simulink model "ardupilot_sil_connector_example"  (R2022a)
settings: Solver=FixedStepAuto  StartTime=0.0  StopTime=inf  FixedStep=0.01  RelTol=1e-3
settings Model: Creator=kboychev  LastModifiedBy=kboychev
settings SolverCC: AlgebraicLoopSolver=TrustRegion
settings DataIOCC: ReturnWorkspaceOutputs=off
settings DebuggingCC: UnconnectedInputMsg=warning  UnconnectedOutputMsg=warning  UnconnectedLineMsg=warning  SFMachineParentedDataDiag=warning  ArithmeticOperatorsInVariantConditions=warning
settings SFSimCC: CustomCodeUndefinedFunction=UseInterfaceOnly

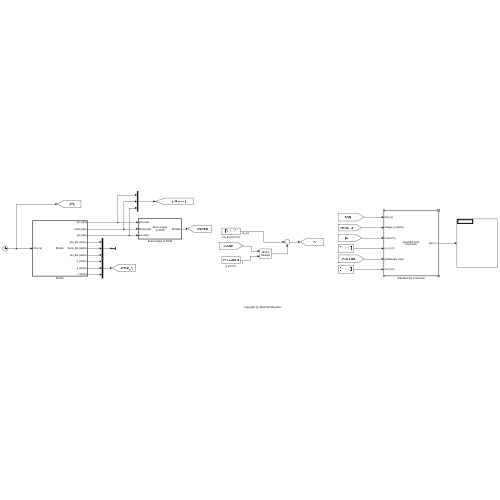
[thumbnail: Simulink's stored preview of the top-level diagram]
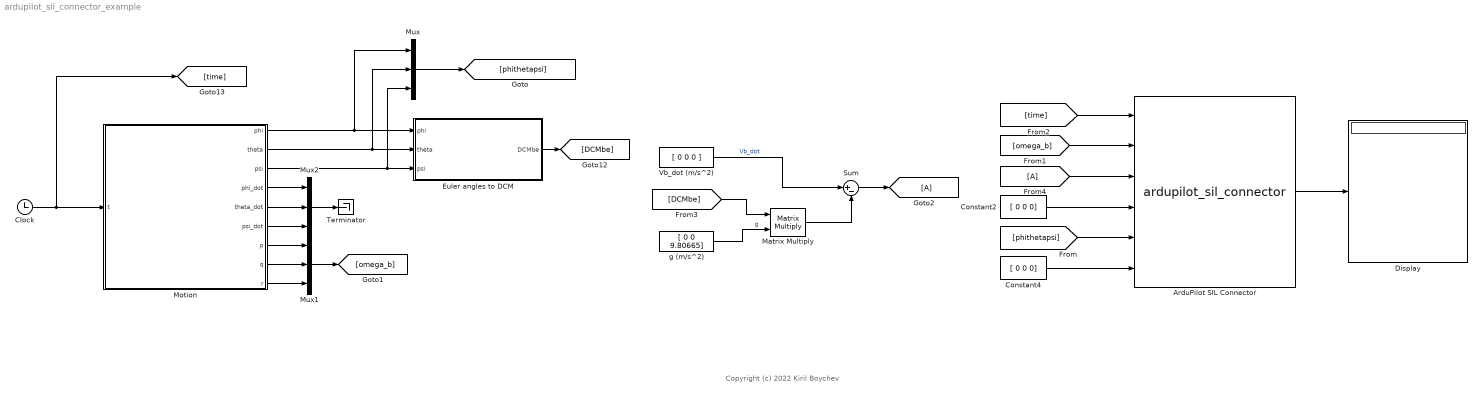
== system ardupilot_sil_connector_example ==
  note: Copyright (c) 2022 Kiril Boychev
  ArduPilot SIL Connector : S-Function  FunctionName=ardupilot_sil_connector  SFunctionDeploymentMode=off  EnableBusSupport=off
      mask Display:
      | fprintf('ArduPilot SITL\nConnector');
      | port_label('input', 1, 'time (s)');
      | port_label('input', 2, 'omega_b (rad/s)');
      | port_label('input', 3, 'A (m/s^2)');
      | port_label('input', 4, 'x y z (m)');
      | port_label('input', 5, 'phithetapsi (rad)');
      | port_label('input', 6, 'Vb (m/s)');
      | port_label('output', 1, 'pwm (-)');
  Clock : Clock
  Constant2 : Constant  Value=[ 0 0 0]
  Constant4 : Constant  Value=[ 0 0 0]
  Display : Display
  Euler angles to DCM : MATLAB Function  TreatAsAtomicUnit=on
  From4 : From
  Goto2 : Goto
  Matrix Multiply : Product  Multiplication=Matrix(*)
  Motion : MATLAB Function  TreatAsAtomicUnit=on
  Mux : Mux  Inputs=3
  Mux1 : Mux  Inputs=3
  Mux2 : Mux  Inputs=3
  Sum : Sum  Inputs=|+-
  Terminator : Terminator
  Vb_dot (m/s^2) : Constant  Value=[ 0 0 0 ]
  g (m/s^2) : Constant  Value=[ 0 0 9.80665]
  wires:
  ArduPilot SIL Connector/1 -> Display/1
  Constant2/1 -> ArduPilot SIL Connector/4
  [phithetapsi] -> ArduPilot SIL Connector/5
  [omega_b] -> ArduPilot SIL Connector/2
  [time] -> ArduPilot SIL Connector/1
  Motion/1(phi) -> Euler angles to DCM/1(phi), Mux/1
  Motion/3(psi) -> Mux/3, Euler angles to DCM/3(psi)
  Motion/2(theta) -> Mux/2, Euler angles to DCM/2(theta)
  Motion/7(p) -> Mux1/1
  Clock/1 -> [time], Motion/1(t)
  Mux/1 -> [phithetapsi]
  Mux1/1 -> [omega_b]
  Euler angles to DCM/1(DCMbe) -> [DCMbe]
  Motion/4(phi_dot) -> Mux2/1
  Motion/9(r) -> Mux1/3
  Mux2/1 -> Terminator/1
  Motion/5(theta_dot) -> Mux2/2
  Motion/8(q) -> Mux1/2
  Motion/6(psi_dot) -> Mux2/3
  Constant4/1 -> ArduPilot SIL Connector/6
  [DCMbe] -> Matrix Multiply/1
  g (m/s^2)/1 -> Matrix Multiply/2  "g"
  Matrix Multiply/1 -> Sum/2
  Vb_dot (m/s^2)/1 -> Sum/1  "Vb_dot"
  From4/1 -> ArduPilot SIL Connector/3
  Sum/1 -> Goto2/1

== matlab function ardupilot_sil_connector_example/Motion ==
  data: t input; phi output; theta output; psi output; phi_dot output; theta_dot output; psi_dot output; p output; q output; r output
function [phi,theta,psi,phi_dot,theta_dot,psi_dot,p,q,r] = motion(t)

phi=0;
theta=0;
psi=0;
phi_dot=0;
theta_dot=0;
psi_dot=0;
p=0;
q=0;
r=0;

if t > 60 %simulate sinusoidal motion after 60s
    
    phi=deg2rad(10)*sin(0.5*t);
    phi_dot=deg2rad(10)*cos(0.5*t)*0.5;
    theta=deg2rad(15)*sin(1*t);
    theta_dot=deg2rad(15)*cos(1*t)*1;
    psi=deg2rad(5)*sin(1.5*t);
    psi_dot=deg2rad(5)*cos(1.5*t)*1.5;

    sphi=sin(phi);
    cphi=cos(phi);
    stheta=sin(theta);
    ctheta=cos(theta);

    pqr=[1,sphi*stheta/ctheta,cphi*stheta/ctheta;
        0,cphi,-sphi;
        0,sphi/ctheta,cphi/ctheta]\[phi_dot;theta_dot;psi_dot];
    
    p=pqr(1);
    q=pqr(2);
    r=pqr(3);

end

== matlab function ardupilot_sil_connector_example/Euler angles to DCM ==
  data: phi input; DCMbe output; theta input; psi input
function DCMbe = DCMeb(phi,theta,psi)

S_phi=sin(phi);
C_phi=cos(phi);
S_theta=sin(theta);
C_theta=cos(theta);
S_psi=sin(psi);
C_psi=cos(psi);

DCMbe=zeros(3,3);

DCMbe(1,1)=C_theta*C_psi;
DCMbe(1,2)=C_theta*S_psi;
DCMbe(1,3)=-S_theta;

DCMbe(2,1)=S_phi*S_theta*C_psi-C_phi*S_psi;
DCMbe(2,2)=S_phi*S_theta*S_psi+C_phi*C_psi;
DCMbe(2,3)=S_phi*C_theta;

DCMbe(3,1)=C_phi*S_theta*C_psi+S_phi*S_psi;
DCMbe(3,2)=C_phi*S_theta*S_psi-S_phi*C_psi;
DCMbe(3,3)=C_phi*C_theta;
